simulink model "sequentialProcessorNarenKolli"  (R2018b)
settings: Solver=VariableStepAuto  StartTime=0.0  StopTime=10  RelTol=1e-3
libraries: hdlsllib x172, simulink_extras x9
(part 1 of 4)
settings Model: Creator=User  LastModifiedBy=kolli
settings DataIOCC: ReturnWorkspaceOutputs=on

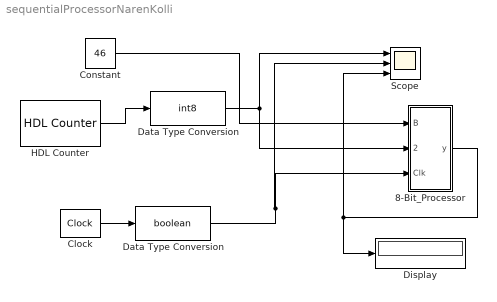
== system sequentialProcessorNarenKolli ==
  "8-Bit_Processor " : Subsystem
  "Clock " : simulink_extras/Flip Flops/Clock  period=1
  "Constant " : Constant  Value=46  OutDataTypeStr=uint8  SampleTime=1
  "Data Type Conversion " : DataTypeConversion  OutDataTypeStr=boolean
  "Data Type Conversion " : DataTypeConversion  OutDataTypeStr=int8
  "Display " : Display
  "HDL Counter " : hdlsllib/Sources/HDL Counter  CountType=Free running  CountInit=0  CountStep=1  CountMax=25  CountFromType=Initial value  CountFrom=0  CountResetPort=off  CountLoadPort=off  CountEnbPort=off  CountDirPort=off  CountDataType=Unsigned  CountWordLen=2  CountFracLen=0  CountSampTime=1
      settings: SourceProductName=Simulink
  "Scope " : Scope  NumInputPorts=3
  wires:
  "Constant "/1 -> "8-Bit_Processor "/1(B)
  "Data Type Conversion "/1 -> "Scope "/2, "8-Bit_Processor "/3("Clk ")
  "Clock "/1 -> "Data Type Conversion "/1
  "8-Bit_Processor "/1(y) -> "Scope "/3, "Display "/1
  "HDL Counter "/1 -> "Data Type Conversion "/1
  "Data Type Conversion "/1 -> "8-Bit_Processor "/2(Code), "Scope "/1

== system sequentialProcessorNarenKolli/8-Bit_Processor  ==
  B : Inport
  Code : Inport  Port=2
  "Clk " : Inport  Port=3
  8-Bit_Adder : Subsystem
  8-Bit_Bitwise_AND : Subsystem
  8-Bit_Multiplier : Subsystem
  8-Bit_Subtractor : Subsystem
  8-bit 4-to-1 MUX : Subsystem
  8-bit Register : Subsystem
  y : Outport  VectorParamsAs1DForOutWhenUnconnected=on
  wires:
  Code/1 -> 8-bit 4-to-1 MUX/1(s)
  8-bit 4-to-1 MUX/1(Y) -> 8-bit Register/1(Data_In), y/1
  8-Bit_Bitwise_AND/1(Y) -> 8-bit 4-to-1 MUX/5(D(11))
  "Clk "/1 -> 8-bit Register/2(Clk)
  8-Bit_Subtractor/1(Diff) -> 8-bit 4-to-1 MUX/4(C(10))
  8-bit Register/1(Y) -> 8-Bit_Bitwise_AND/2(B), 8-Bit_Subtractor/1(A), 8-Bit_Adder/2("B "), 8-Bit_Multiplier/2(B)
  8-Bit_Adder/1(Sum) -> 8-bit 4-to-1 MUX/2(A(00))
  8-Bit_Multiplier/1(Product) -> 8-bit 4-to-1 MUX/3(B(01))
  B/1 -> 8-Bit_Multiplier/1(A), 8-Bit_Adder/1("A "), 8-Bit_Bitwise_AND/1(A), 8-Bit_Subtractor/2(B)

== system sequentialProcessorNarenKolli/8-Bit_Processor /8-Bit_Adder ==
  "A " : Inport  OutDataTypeStr=uint8
  "B " : Inport  Port=2  OutDataTypeStr=uint8
  "Bit Concat " : hdlsllib/Logic and Bit Operations/Bit Concat  numInputs=8
      settings: SourceProductName=HDL Coder  SourceProductBaseCode=HD
  Constant2 : Constant  Value=0  OutDataTypeStr=boolean
  "Full Adder 0 " : Subsystem
  "Full Adder 1 " : Subsystem
  "Full Adder 2 " : Subsystem
  "Full Adder 3 " : Subsystem
  "Full Adder 4 " : Subsystem
  "Full Adder 5 " : Subsystem
  "Full Adder 6 " : Subsystem
  "Full Adder 7 " : Subsystem
  "Slicer1 " : Subsystem
  "Slicer2 " : Subsystem
  Sum : Outport  OutDataTypeStr=uint8
  wires:
  "Slicer1 "/3(Y5) -> "Full Adder 2 "/1(X)
  "Slicer2 "/7(Y1) -> "Full Adder 6 "/2(Y)
  "Full Adder 0 "/1(S) -> "Bit Concat "/1
  "Slicer1 "/1(Y7) -> "Full Adder 0 "/1(X)
  "Full Adder 1 "/1(S) -> "Bit Concat "/2
  "Slicer1 "/2(Y6) -> "Full Adder 1 "/1(X)
  "Slicer1 "/7(Y1) -> "Full Adder 6 "/1(X)
  "Slicer2 "/3(Y5) -> "Full Adder 2 "/2(Y)
  "Full Adder 5 "/1(S) -> "Bit Concat "/6
  "Slicer2 "/4(Y4) -> "Full Adder 3 "/2(Y)
  "Full Adder 3 "/2(C) -> "Full Adder 2 "/3(Z)
  "Full Adder 6 "/2(C) -> "Full Adder 5 "/3(Z)
  "Slicer1 "/6(Y2) -> "Full Adder 5 "/1(X)
  "B "/1 -> "Slicer2 "/1(X)
  "Slicer1 "/8(Y0) -> "Full Adder 7 "/1(X)
  "Full Adder 7 "/1(S) -> "Bit Concat "/8
  "Full Adder 6 "/1(S) -> "Bit Concat "/7
  "Slicer2 "/1(Y7) -> "Full Adder 0 "/2(Y)
  "Full Adder 3 "/1(S) -> "Bit Concat "/4
  "Full Adder 4 "/1(S) -> "Bit Concat "/5
  "Full Adder 2 "/2(C) -> "Full Adder 1 "/3(Z)
  "Slicer2 "/8(Y0) -> "Full Adder 7 "/2(Y)
  "Slicer2 "/2(Y6) -> "Full Adder 1 "/2(Y)
  "Full Adder 2 "/1(S) -> "Bit Concat "/3
  "Full Adder 7 "/2(C) -> "Full Adder 6 "/3(Z)
  Constant2/1 -> "Full Adder 7 "/3(Z)
  "Full Adder 1 "/2(C) -> "Full Adder 0 "/3(Z)
  "Full Adder 4 "/2(C) -> "Full Adder 3 "/3(Z)
  "Bit Concat "/1 -> Sum/1
  "Slicer2 "/6(Y2) -> "Full Adder 5 "/2(Y)
  "Slicer2 "/5(Y3) -> "Full Adder 4 "/2(Y)
  "A "/1 -> "Slicer1 "/1(X)
  "Full Adder 5 "/2(C) -> "Full Adder 4 "/3(Z)
  "Slicer1 "/4(Y4) -> "Full Adder 3 "/1(X)
  "Slicer1 "/5(Y3) -> "Full Adder 4 "/1(X)

== system sequentialProcessorNarenKolli/8-Bit_Processor /8-Bit_Bitwise_AND ==
  A : Inport
  B : Inport  Port=2
  AND{,1..7} (8 alike) : Logic  AllPortsSameDT=off  OutDataTypeStr=boolean
  Bit Concat Block : hdlsllib/Logic and Bit Operations/Bit Concat  numInputs=8
      settings: SourceProductName=HDL Coder  SourceProductBaseCode=HD
  First Bit Slicer : Subsystem
  Second Bit Slicer : Subsystem
  Y : Outport
  wires:
  AND2/1 -> Bit Concat Block/6
  AND4/1 -> Bit Concat Block/4
  Bit Concat Block/1 -> Y/1
  AND7/1 -> Bit Concat Block/1
  AND3/1 -> Bit Concat Block/5
  AND6/1 -> Bit Concat Block/2
  First Bit Slicer/6(Y2) -> AND2/1
  Second Bit Slicer/6(Y2) -> AND2/2
  Second Bit Slicer/1(Y7) -> AND7/2
  Second Bit Slicer/8(Y0) -> AND/2
  AND1/1 -> Bit Concat Block/7
  First Bit Slicer/7(Y1) -> AND1/1
  A/1 -> First Bit Slicer/1(X)
  B/1 -> Second Bit Slicer/1(X)
  Second Bit Slicer/7(Y1) -> AND1/2
  AND5/1 -> Bit Concat Block/3
  First Bit Slicer/8(Y0) -> AND/1
  First Bit Slicer/5(Y3) -> AND3/1
  AND/1 -> Bit Concat Block/8
  Second Bit Slicer/5(Y3) -> AND3/2
  Second Bit Slicer/4(Y4) -> AND4/2
  Second Bit Slicer/3(Y5) -> AND5/2
  First Bit Slicer/3(Y5) -> AND5/1
  First Bit Slicer/2(Y6) -> AND6/1
  First Bit Slicer/4(Y4) -> AND4/1
  Second Bit Slicer/2(Y6) -> AND6/2
  First Bit Slicer/1(Y7) -> AND7/1

== system sequentialProcessorNarenKolli/8-Bit_Processor /8-Bit_Multiplier ==
  A : Inport  OutDataTypeStr=uint8
  B : Inport  Port=2  OutDataTypeStr=uint8
  "First 4x4 Multiplier " : Subsystem
  First 8-Bit_Adder : Subsystem
  "First Bit Concat " : hdlsllib/Logic and Bit Operations/Bit Concat  numInputs=8
      settings: SourceProductName=HDL Coder  SourceProductBaseCode=HD
  First Constant : Constant  Value=0  OutDataTypeStr=boolean
  "First Slicer " : Subsystem
  "Fourth Bit Concat " : hdlsllib/Logic and Bit Operations/Bit Concat  numInputs=8
      settings: SourceProductName=HDL Coder  SourceProductBaseCode=HD
  Fourth Constant : Constant  Value=0  OutDataTypeStr=boolean
  Second 4x4 Multiplier : Subsystem
  Second 8-Bit_Adder1 : Subsystem
  "Second Bit Concat " : hdlsllib/Logic and Bit Operations/Bit Concat  numInputs=8
      settings: SourceProductName=HDL Coder  SourceProductBaseCode=HD
  Second Constant : Constant  Value=0  OutDataTypeStr=boolean
  Second Slicer : Subsystem
  Third Slicer : Subsystem
  Third 4x4 Multiplier : Subsystem
  "Third Bit Concat " : hdlsllib/Logic and Bit Operations/Bit Concat  numInputs=8
      settings: SourceProductName=HDL Coder  SourceProductBaseCode=HD
  Third Constant : Constant  Value=0  OutDataTypeStr=boolean
  Product : Outport  OutDataTypeStr=uint8
  wires:
  A/1 -> "First Slicer "/1(X)
  "First Slicer "/6(Y2) -> Third 4x4 Multiplier/2(A2), Second 4x4 Multiplier/2(A2)
  Third 4x4 Multiplier/6(Bit-2) -> "Fourth Bit Concat "/6
  "First Slicer "/5(Y3) -> Third 4x4 Multiplier/1(A3), Second 4x4 Multiplier/1(A3)
  Second 4x4 Multiplier/8(Bit-0) -> "Second Bit Concat "/8
  "First 4x4 Multiplier "/6(Bit-2) -> "First Bit Concat "/6
  "Second Bit Concat "/1 -> First 8-Bit_Adder/2(B)
  "First Slicer "/1(Y7) -> "First 4x4 Multiplier "/1(A3)
  Second Slicer/4(Y4) -> Second 4x4 Multiplier/8(B0)
  Second Slicer/1(Y7) -> Second 4x4 Multiplier/5(B3)
  Second Slicer/6(Y2) -> "First 4x4 Multiplier "/6(B2), Third 4x4 Multiplier/6(B2)
  "First Slicer "/7(Y1) -> Third 4x4 Multiplier/3(A1), Second 4x4 Multiplier/3(A1)
  Second Slicer/7(Y1) -> "First 4x4 Multiplier "/7(B1), Third 4x4 Multiplier/7(B1)
  Third Slicer/5(Y3) -> "Fourth Bit Concat "/1
  "First Slicer "/8(Y0) -> Third 4x4 Multiplier/4(A0), Second 4x4 Multiplier/4(A0)
  "Third Bit Concat "/1 -> Second 8-Bit_Adder1/2(B)
  Third Slicer/8(Y0) -> "Fourth Bit Concat "/4
  First 8-Bit_Adder/1(Sum) -> Second 8-Bit_Adder1/1(A)
  Second Slicer/5(Y3) -> Third 4x4 Multiplier/5(B3), "First 4x4 Multiplier "/5(B3)
  "First Slicer "/2(Y6) -> "First 4x4 Multiplier "/2(A2)
  "First 4x4 Multiplier "/7(Bit-1) -> "First Bit Concat "/7
  Second Slicer/8(Y0) -> "First 4x4 Multiplier "/8(B0), Third 4x4 Multiplier/8(B0)
  Third 4x4 Multiplier/1(Bit-7) -> "Third Bit Concat "/5
  Third Constant/1 -> "Third Bit Concat "/3
  "First Slicer "/3(Y5) -> "First 4x4 Multiplier "/3(A1)
  "First Slicer "/4(Y4) -> "First 4x4 Multiplier "/4(A0)
  First Constant/1 -> "Third Bit Concat "/1
  Second Slicer/3(Y5) -> Second 4x4 Multiplier/7(B1)
  Second Slicer/2(Y6) -> Second 4x4 Multiplier/6(B2)
  Third 4x4 Multiplier/8(Bit-0) -> "Fourth Bit Concat "/8
  "First Bit Concat "/1 -> First 8-Bit_Adder/1(A)
  "Fourth Bit Concat "/1 -> Product/1
  Third 4x4 Multiplier/5(Bit-3) -> "Fourth Bit Concat "/5
  Second 4x4 Multiplier/7(Bit-1) -> "Second Bit Concat "/7
  Third Slicer/7(Y1) -> "Fourth Bit Concat "/3
  Second 4x4 Multiplier/3(Bit-5) -> "Second Bit Concat "/3
  Third 4x4 Multiplier/7(Bit-1) -> "Fourth Bit Concat "/7
  Second 8-Bit_Adder1/1(Sum) -> Third Slicer/1(X)
  B/1 -> Second Slicer/1(X)
  Third Slicer/6(Y2) -> "Fourth Bit Concat "/2
  "First 4x4 Multiplier "/2(Bit-6) -> "First Bit Concat "/2
  "First 4x4 Multiplier "/4(Bit-4) -> "First Bit Concat "/4
  "First 4x4 Multiplier "/8(Bit-0) -> "First Bit Concat "/8
  Second 4x4 Multiplier/6(Bit-2) -> "Second Bit Concat "/6
  Second 4x4 Multiplier/5(Bit-3) -> "Second Bit Concat "/5
  Fourth Constant/1 -> "Third Bit Concat "/4
  Second 4x4 Multiplier/4(Bit-4) -> "Second Bit Concat "/4
  "First 4x4 Multiplier "/3(Bit-5) -> "First Bit Concat "/3
  "First 4x4 Multiplier "/5(Bit-3) -> "First Bit Concat "/5
  "First 4x4 Multiplier "/1(Bit-7) -> "First Bit Concat "/1
  Second 4x4 Multiplier/2(Bit-6) -> "Second Bit Concat "/2
  Second Constant/1 -> "Third Bit Concat "/2
  Third 4x4 Multiplier/4(Bit-4) -> "Third Bit Concat "/8
  Third 4x4 Multiplier/3(Bit-5) -> "Third Bit Concat "/7
  Third 4x4 Multiplier/2(Bit-6) -> "Third Bit Concat "/6
  Second 4x4 Multiplier/1(Bit-7) -> "Second Bit Concat "/1

== system sequentialProcessorNarenKolli/8-Bit_Processor /8-Bit_Subtractor ==
  A : Inport  OutDataTypeStr=uint8
  B : Inport  Port=2  OutDataTypeStr=uint8
  Bit Concat : hdlsllib/Logic and Bit Operations/Bit Concat  numInputs=8
      settings: SourceProductName=HDL Coder  SourceProductBaseCode=HD
  Constant2 : Constant  OutDataTypeStr=boolean
  Full Adder 0 : Subsystem
  Full Adder 1 : Subsystem
  "Full Adder 2 " : Subsystem
  "Full Adder 3 " : Subsystem
  Full Adder 4 : Subsystem
  "Full Adder 5 " : Subsystem
  "Full Adder 6 " : Subsystem
  "Full Adder 7 " : Subsystem
  "NOT 0 " : Logic  Operator=NOT  AllPortsSameDT=off  OutDataTypeStr=boolean
  NOT {1..7} (7 alike) : Logic  Operator=NOT  AllPortsSameDT=off  OutDataTypeStr=boolean
  "Slicer 1 " : Subsystem
  "Slicer 2 " : Subsystem
  Diff : Outport  OutDataTypeStr=uint8
  wires:
  "Slicer 1 "/3(Y5) -> "Full Adder 2 "/1(X)
  "Slicer 2 "/7(Y1) -> NOT 6/1
  Full Adder 0/1(S) -> Bit Concat/1
  "Slicer 1 "/1(Y7) -> Full Adder 0/1(X)
  Full Adder 1/1(S) -> Bit Concat/2
  "Slicer 1 "/2(Y6) -> Full Adder 1/1(X)
  "Slicer 1 "/7(Y1) -> "Full Adder 6 "/1(X)
  "Slicer 2 "/3(Y5) -> NOT 2/1
  "Full Adder 5 "/1(S) -> Bit Concat/6
  "Slicer 2 "/4(Y4) -> NOT 3/1
  "Full Adder 3 "/2(C) -> "Full Adder 2 "/3(Z)
  "Full Adder 6 "/2(C) -> "Full Adder 5 "/3(Z)
  "Slicer 1 "/6(Y2) -> "Full Adder 5 "/1(X)
  B/1 -> "Slicer 2 "/1(X)
  "Slicer 1 "/8(Y0) -> "Full Adder 7 "/1(X)
  "Full Adder 7 "/1(S) -> Bit Concat/8
  "Full Adder 6 "/1(S) -> Bit Concat/7
  "NOT 0 "/1 -> Full Adder 0/2(Y)
  "Full Adder 3 "/1(S) -> Bit Concat/4
  Full Adder 4/1(S) -> Bit Concat/5
  "Full Adder 2 "/2(C) -> Full Adder 1/3(Z)
  "Slicer 2 "/8(Y0) -> NOT 7/1
  "Slicer 2 "/2(Y6) -> NOT 1/1
  "Full Adder 2 "/1(S) -> Bit Concat/3
  "Full Adder 7 "/2(C) -> "Full Adder 6 "/3(Z)
  Constant2/1 -> "Full Adder 7 "/3(Z)
  Full Adder 1/2(C) -> Full Adder 0/3(Z)
  Full Adder 4/2(C) -> "Full Adder 3 "/3(Z)
  Bit Concat/1 -> Diff/1
  "Slicer 2 "/6(Y2) -> NOT 5/1
  "Slicer 2 "/5(Y3) -> NOT 4/1
  A/1 -> "Slicer 1 "/1(X)
  "Full Adder 5 "/2(C) -> Full Adder 4/3(Z)
  "Slicer 1 "/4(Y4) -> "Full Adder 3 "/1(X)
  "Slicer 1 "/5(Y3) -> Full Adder 4/1(X)
  NOT 1/1 -> Full Adder 1/2(Y)
  "Slicer 2 "/1(Y7) -> "NOT 0 "/1
  NOT 2/1 -> "Full Adder 2 "/2(Y)
  NOT 3/1 -> "Full Adder 3 "/2(Y)
  NOT 4/1 -> Full Adder 4/2(Y)
  NOT 5/1 -> "Full Adder 5 "/2(Y)
  NOT 6/1 -> "Full Adder 6 "/2(Y)
  NOT 7/1 -> "Full Adder 7 "/2(Y)

== system sequentialProcessorNarenKolli/8-Bit_Processor /8-bit 4-to-1 MUX ==
  s : Inport
  A(00) : Inport  Port=2
  B(01) : Inport  Port=3
  C(10) : Inport  Port=4
  D(11) : Inport  Port=5
  4 x 1 MUX : Subsystem
  4 x 1 MUX1 : Subsystem
  4 x 1 MUX2 : Subsystem
  4 x 1 MUX3 : Subsystem
  4 x 1 MUX4 : Subsystem
  4 x 1 MUX5 : Subsystem
  4 x 1 MUX6 : Subsystem
  4 x 1 MUX7 : Subsystem
  Bit Concat : hdlsllib/Logic and Bit Operations/Bit Concat  numInputs=8
      settings: SourceProductName=Simulink
  Slicer : Subsystem
  Slicer1 : Subsystem
  Slicer2 : Subsystem
  Slicer3 : Subsystem
  Y : Outport  VectorParamsAs1DForOutWhenUnconnected=on
  wires:
  Slicer1/7(Y6) -> 4 x 1 MUX6/4(x1)
  Slicer3/8(Y7) -> 4 x 1 MUX7/5(x3)
  Slicer1/8(Y7) -> 4 x 1 MUX7/4(x1)
  s/1 -> 4 x 1 MUX/1(s), 4 x 1 MUX6/1(s), 4 x 1 MUX7/1(s), 4 x 1 MUX5/1(s), 4 x 1 MUX4/1(s), 4 x 1 MUX3/1(s), 4 x 1 MUX2/1(s), 4 x 1 MUX1/1(s)
  A(00)/1 -> Slicer/1(In1)
  Slicer/8(Y7) -> 4 x 1 MUX7/2("x0 ")
  Slicer2/1(Y0) -> 4 x 1 MUX/3(x2)
  4 x 1 MUX5/1(y) -> Bit Concat/3
  Bit Concat/1 -> Y/1
  Slicer3/2(Y1) -> 4 x 1 MUX1/5(x3)
  Slicer/7(Y6) -> 4 x 1 MUX6/2("x0 ")
  D(11)/1 -> Slicer3/1(In1)
  Slicer2/6(Y5) -> 4 x 1 MUX5/3(x2)
  4 x 1 MUX7/1(y) -> Bit Concat/1
  Slicer3/3(Y2) -> 4 x 1 MUX2/5(x3)
  Slicer3/5(Y4) -> 4 x 1 MUX4/5(x3)
  Slicer/6(Y5) -> 4 x 1 MUX5/2("x0 ")
  B(01)/1 -> Slicer1/1(In1)
  Slicer3/6(Y5) -> 4 x 1 MUX5/5(x3)
  Slicer3/7(Y6) -> 4 x 1 MUX6/5(x3)
  Slicer2/5(Y4) -> 4 x 1 MUX4/3(x2)
  Slicer2/2(Y1) -> 4 x 1 MUX1/3(x2)
  4 x 1 MUX/1(y) -> Bit Concat/8
  4 x 1 MUX4/1(y) -> Bit Concat/4
  4 x 1 MUX3/1(y) -> Bit Concat/5
  4 x 1 MUX6/1(y) -> Bit Concat/2
  Slicer1/3(Y2) -> 4 x 1 MUX2/4(x1)
  Slicer2/3(Y2) -> 4 x 1 MUX2/3(x2)
  Slicer1/6(Y5) -> 4 x 1 MUX5/4(x1)
  Slicer1/4(Y3) -> 4 x 1 MUX3/4(x1)
  Slicer2/8(Y7) -> 4 x 1 MUX7/3(x2)
  Slicer/2(Y1) -> 4 x 1 MUX1/2("x0 ")
  Slicer/4(Y3) -> 4 x 1 MUX3/2("x0 ")
  Slicer2/4(Y3) -> 4 x 1 MUX3/3(x2)
  Slicer3/1(Y0) -> 4 x 1 MUX/5(x3)
  Slicer3/4(Y3) -> 4 x 1 MUX3/5(x3)
  Slicer1/5(Y4) -> 4 x 1 MUX4/4(x1)
  Slicer/3(Y2) -> 4 x 1 MUX2/2("x0 ")
  Slicer/5(Y4) -> 4 x 1 MUX4/2("x0 ")
  Slicer2/7(Y6) -> 4 x 1 MUX6/3(x2)
  4 x 1 MUX1/1(y) -> Bit Concat/7
  Slicer1/2(Y1) -> 4 x 1 MUX1/4(x1)
  C(10)/1 -> Slicer2/1(In1)
  Slicer1/1(Y0) -> 4 x 1 MUX/4(x1)
  4 x 1 MUX2/1(y) -> Bit Concat/6
  Slicer/1(Y0) -> 4 x 1 MUX/2("x0 ")

== system sequentialProcessorNarenKolli/8-Bit_Processor /8-bit Register ==
  Data_In : Inport
  Clk : Inport  Port=2
  Bit Concat : hdlsllib/Logic and Bit Operations/Bit Concat  numInputs=8
      settings: SourceProductName=Simulink
  Constant : Constant  OutDataTypeStr=boolean  SampleTime=1
  D Flip-Flop{,1..7} (8 alike) : simulink_extras/Flip Flops/D Flip-Flop
      settings: SourceProductName=Simulink
  Slicer : Subsystem
  Terminator{,1..7} (8 alike) : Terminator
  Y : Outport  VectorParamsAs1DForOutWhenUnconnected=on
  wires:
  Constant/1 -> D Flip-Flop4/3, D Flip-Flop7/3, D Flip-Flop6/3, D Flip-Flop5/3, D Flip-Flop3/3, D Flip-Flop2/3, D Flip-Flop1/3, D Flip-Flop/3
  Clk/1 -> D Flip-Flop6/2, D Flip-Flop7/2, D Flip-Flop5/2, D Flip-Flop4/2, D Flip-Flop3/2, D Flip-Flop2/2, D Flip-Flop1/2, D Flip-Flop/2
  D Flip-Flop5/1 -> Bit Concat/3
  Slicer/8(Y7) -> D Flip-Flop7/1
  D Flip-Flop1/2 -> Terminator1/1
  D Flip-Flop/1 -> Bit Concat/8
  D Flip-Flop1/1 -> Bit Concat/7
  Data_In/1 -> Slicer/1(In1)
  D Flip-Flop2/2 -> Terminator2/1
  Bit Concat/1 -> Y/1
  Slicer/7(Y6) -> D Flip-Flop6/1
  D Flip-Flop7/1 -> Bit Concat/1
  D Flip-Flop6/2 -> Terminator6/1
  D Flip-Flop4/2 -> Terminator4/1
  Slicer/4(Y3) -> D Flip-Flop3/1
  D Flip-Flop3/2 -> Terminator3/1
  D Flip-Flop2/1 -> Bit Concat/6
  Slicer/2(Y1) -> D Flip-Flop1/1
  D Flip-Flop/2 -> Terminator/1
  D Flip-Flop4/1 -> Bit Concat/4
  D Flip-Flop7/2 -> Terminator7/1
  D Flip-Flop3/1 -> Bit Concat/5
  Slicer/5(Y4) -> D Flip-Flop4/1
  Slicer/1(Y0) -> D Flip-Flop/1
  D Flip-Flop5/2 -> Terminator5/1
  Slicer/6(Y5) -> D Flip-Flop5/1
  Slicer/3(Y2) -> D Flip-Flop2/1
  D Flip-Flop6/1 -> Bit Concat/2

== system sequentialProcessorNarenKolli/8-Bit_Processor /8-Bit_Adder/Full Adder 0  ==
  X : Inport
  Y : Inport  Port=2
  Z : Inport  Port=3
  Half Adder : Subsystem
  Half Adder1 : Subsystem
  OR : Logic  Operator=OR  AllPortsSameDT=off  OutDataTypeStr=boolean
  S : Outport
  C : Outport  Port=2
  wires:
  Half Adder/2(Carry) -> OR/2
  OR/1 -> C/1
  Z/1 -> Half Adder1/2(B)
  X/1 -> Half Adder/1(A)
  Half Adder1/1(Sum) -> S/1
  Half Adder/1(Sum) -> Half Adder1/1(A)
  Y/1 -> Half Adder/2(B)
  Half Adder1/2(Carry) -> OR/1

== system sequentialProcessorNarenKolli/8-Bit_Processor /8-Bit_Adder/Full Adder 1  ==
  X : Inport
  Y : Inport  Port=2
  Z : Inport  Port=3
  Half Adder : Subsystem
  Half Adder1 : Subsystem
  OR : Logic  Operator=OR  AllPortsSameDT=off  OutDataTypeStr=boolean
  S : Outport
  C : Outport  Port=2
  wires:
  Half Adder/2(Carry) -> OR/2
  OR/1 -> C/1
  Z/1 -> Half Adder1/2(B)
  X/1 -> Half Adder/1(A)
  Half Adder1/1(Sum) -> S/1
  Half Adder/1(Sum) -> Half Adder1/1(A)
  Y/1 -> Half Adder/2(B)
  Half Adder1/2(Carry) -> OR/1

== system sequentialProcessorNarenKolli/8-Bit_Processor /8-Bit_Adder/Full Adder 2  ==
  X : Inport
  Y : Inport  Port=2
  Z : Inport  Port=3
  Half Adder : Subsystem
  Half Adder1 : Subsystem
  OR : Logic  Operator=OR  AllPortsSameDT=off  OutDataTypeStr=boolean
  S : Outport
  C : Outport  Port=2
  wires:
  Half Adder/2(Carry) -> OR/2
  OR/1 -> C/1
  Z/1 -> Half Adder1/2(B)
  X/1 -> Half Adder/1(A)
  Half Adder1/1(Sum) -> S/1
  Half Adder/1(Sum) -> Half Adder1/1(A)
  Y/1 -> Half Adder/2(B)
  Half Adder1/2(Carry) -> OR/1

== system sequentialProcessorNarenKolli/8-Bit_Processor /8-Bit_Adder/Full Adder 3  ==
  X : Inport
  Y : Inport  Port=2
  Z : Inport  Port=3
  Half Adder : Subsystem
  Half Adder1 : Subsystem
  OR : Logic  Operator=OR  AllPortsSameDT=off  OutDataTypeStr=boolean
  S : Outport
  C : Outport  Port=2
  wires:
  Half Adder/2(Carry) -> OR/2
  OR/1 -> C/1
  Z/1 -> Half Adder1/2(B)
  X/1 -> Half Adder/1(A)
  Half Adder1/1(Sum) -> S/1
  Half Adder/1(Sum) -> Half Adder1/1(A)
  Y/1 -> Half Adder/2(B)
  Half Adder1/2(Carry) -> OR/1

== system sequentialProcessorNarenKolli/8-Bit_Processor /8-Bit_Adder/Full Adder 4  ==
  X : Inport
  Y : Inport  Port=2
  Z : Inport  Port=3
  Half Adder : Subsystem
  Half Adder1 : Subsystem
  OR : Logic  Operator=OR  AllPortsSameDT=off  OutDataTypeStr=boolean
  S : Outport
  C : Outport  Port=2
  wires:
  Half Adder/2(Carry) -> OR/2
  OR/1 -> C/1
  Z/1 -> Half Adder1/2(B)
  X/1 -> Half Adder/1(A)
  Half Adder1/1(Sum) -> S/1
  Half Adder/1(Sum) -> Half Adder1/1(A)
  Y/1 -> Half Adder/2(B)
  Half Adder1/2(Carry) -> OR/1

== system sequentialProcessorNarenKolli/8-Bit_Processor /8-Bit_Adder/Full Adder 5  ==
  X : Inport
  Y : Inport  Port=2
  Z : Inport  Port=3
  Half Adder : Subsystem
  Half Adder1 : Subsystem
  OR : Logic  Operator=OR  AllPortsSameDT=off  OutDataTypeStr=boolean
  S : Outport
  C : Outport  Port=2
  wires:
  Half Adder/2(Carry) -> OR/2
  OR/1 -> C/1
  Z/1 -> Half Adder1/2(B)
  X/1 -> Half Adder/1(A)
  Half Adder1/1(Sum) -> S/1
  Half Adder/1(Sum) -> Half Adder1/1(A)
  Y/1 -> Half Adder/2(B)
  Half Adder1/2(Carry) -> OR/1

== system sequentialProcessorNarenKolli/8-Bit_Processor /8-Bit_Adder/Full Adder 6  ==
  X : Inport
  Y : Inport  Port=2
  Z : Inport  Port=3
  Half Adder : Subsystem
  Half Adder1 : Subsystem
  OR : Logic  Operator=OR  AllPortsSameDT=off  OutDataTypeStr=boolean
  S : Outport
  C : Outport  Port=2
  wires:
  Half Adder/2(Carry) -> OR/2
  OR/1 -> C/1
  Z/1 -> Half Adder1/2(B)
  X/1 -> Half Adder/1(A)
  Half Adder1/1(Sum) -> S/1
  Half Adder/1(Sum) -> Half Adder1/1(A)
  Y/1 -> Half Adder/2(B)
  Half Adder1/2(Carry) -> OR/1

== system sequentialProcessorNarenKolli/8-Bit_Processor /8-Bit_Adder/Full Adder 7  ==
  X : Inport
  Y : Inport  Port=2
  Z : Inport  Port=3
  Half Adder : Subsystem
  Half Adder1 : Subsystem
  OR : Logic  Operator=OR  AllPortsSameDT=off  OutDataTypeStr=boolean
  S : Outport
  C : Outport  Port=2
  wires:
  Half Adder/2(Carry) -> OR/2
  OR/1 -> C/1
  Z/1 -> Half Adder1/2(B)
  X/1 -> Half Adder/1(A)
  Half Adder1/1(Sum) -> S/1
  Half Adder/1(Sum) -> Half Adder1/1(A)
  Y/1 -> Half Adder/2(B)
  Half Adder1/2(Carry) -> OR/1

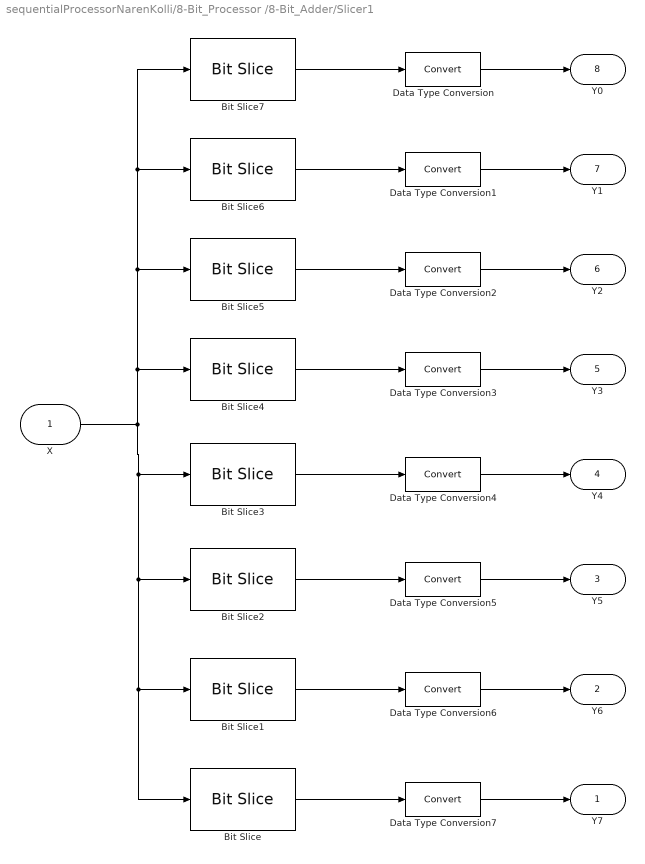
== system sequentialProcessorNarenKolli/8-Bit_Processor /8-Bit_Adder/Slicer1  ==
  X : Inport  OutDataTypeStr=uint8  SampleTime=1
  Bit Slice : hdlsllib/Logic and Bit Operations/Bit Slice  lidx=7  ridx=7
  Bit Slice1 : hdlsllib/Logic and Bit Operations/Bit Slice  lidx=6  ridx=6
  Bit Slice2 : hdlsllib/Logic and Bit Operations/Bit Slice  lidx=5  ridx=5
  Bit Slice3 : hdlsllib/Logic and Bit Operations/Bit Slice  lidx=4  ridx=4
  Bit Slice4 : hdlsllib/Logic and Bit Operations/Bit Slice  lidx=3  ridx=3
  Bit Slice5 : hdlsllib/Logic and Bit Operations/Bit Slice  lidx=2  ridx=2
  Bit Slice6 : hdlsllib/Logic and Bit Operations/Bit Slice  lidx=1  ridx=1
  Bit Slice7 : hdlsllib/Logic and Bit Operations/Bit Slice  lidx=0  ridx=0
  Data Type Conversion{,1..7} (8 alike) : DataTypeConversion
  Y7 : Outport
  Y6 : Outport  Port=2
  Y5 : Outport  Port=3
  Y4 : Outport  Port=4
  Y3 : Outport  Port=5
  Y2 : Outport  Port=6
  Y1 : Outport  Port=7
  Y0 : Outport  Port=8
  wires:
  Data Type Conversion4/1 -> Y4/1
  Bit Slice3/1 -> Data Type Conversion4/1
  X/1 -> Bit Slice3/1, Bit Slice2/1, Bit Slice1/1, Bit Slice/1, Bit Slice4/1, Bit Slice5/1, Bit Slice6/1, Bit Slice7/1
  Bit Slice1/1 -> Data Type Conversion6/1
  Data Type Conversion1/1 -> Y1/1
  Bit Slice6/1 -> Data Type Conversion1/1
  Bit Slice5/1 -> Data Type Conversion2/1
  Bit Slice2/1 -> Data Type Conversion5/1
  Data Type Conversion/1 -> Y0/1
  Bit Slice4/1 -> Data Type Conversion3/1
  Bit Slice/1 -> Data Type Conversion7/1
  Data Type Conversion7/1 -> Y7/1
  Bit Slice7/1 -> Data Type Conversion/1
  Data Type Conversion3/1 -> Y3/1
  Data Type Conversion5/1 -> Y5/1
  Data Type Conversion6/1 -> Y6/1
  Data Type Conversion2/1 -> Y2/1

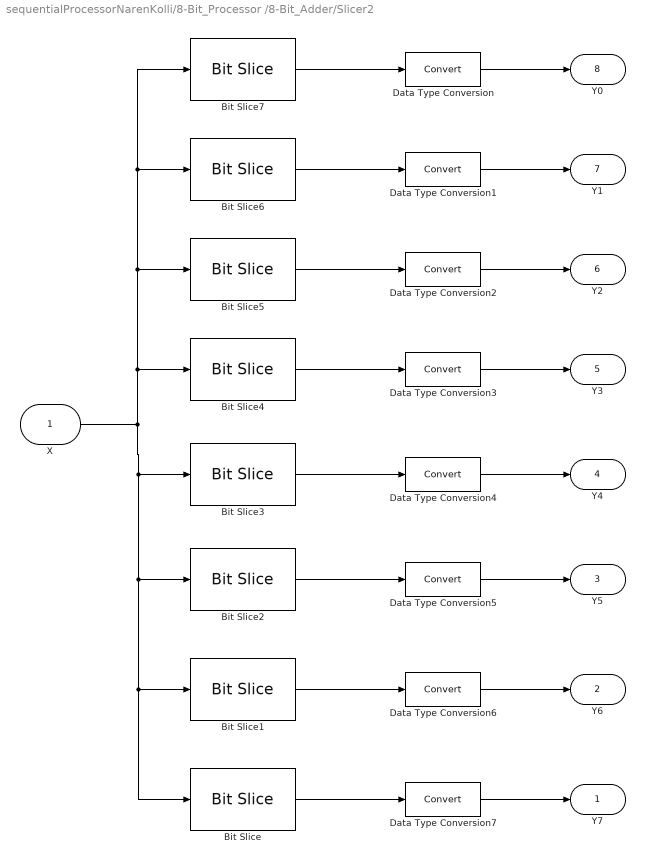
== system sequentialProcessorNarenKolli/8-Bit_Processor /8-Bit_Adder/Slicer2  ==
  X : Inport  OutDataTypeStr=uint8  SampleTime=1
  Bit Slice : hdlsllib/Logic and Bit Operations/Bit Slice  lidx=7  ridx=7
  Bit Slice1 : hdlsllib/Logic and Bit Operations/Bit Slice  lidx=6  ridx=6
  Bit Slice2 : hdlsllib/Logic and Bit Operations/Bit Slice  lidx=5  ridx=5
  Bit Slice3 : hdlsllib/Logic and Bit Operations/Bit Slice  lidx=4  ridx=4
  Bit Slice4 : hdlsllib/Logic and Bit Operations/Bit Slice  lidx=3  ridx=3
  Bit Slice5 : hdlsllib/Logic and Bit Operations/Bit Slice  lidx=2  ridx=2
  Bit Slice6 : hdlsllib/Logic and Bit Operations/Bit Slice  lidx=1  ridx=1
  Bit Slice7 : hdlsllib/Logic and Bit Operations/Bit Slice  lidx=0  ridx=0
  Data Type Conversion{,1..7} (8 alike) : DataTypeConversion
  Y7 : Outport
  Y6 : Outport  Port=2
  Y5 : Outport  Port=3
  Y4 : Outport  Port=4
  Y3 : Outport  Port=5
  Y2 : Outport  Port=6
  Y1 : Outport  Port=7
  Y0 : Outport  Port=8
  wires:
  Data Type Conversion4/1 -> Y4/1
  Bit Slice3/1 -> Data Type Conversion4/1
  X/1 -> Bit Slice3/1, Bit Slice2/1, Bit Slice1/1, Bit Slice/1, Bit Slice4/1, Bit Slice5/1, Bit Slice6/1, Bit Slice7/1
  Bit Slice1/1 -> Data Type Conversion6/1
  Data Type Conversion1/1 -> Y1/1
  Bit Slice6/1 -> Data Type Conversion1/1
  Bit Slice5/1 -> Data Type Conversion2/1
  Bit Slice2/1 -> Data Type Conversion5/1
  Data Type Conversion/1 -> Y0/1
  Bit Slice4/1 -> Data Type Conversion3/1
  Bit Slice/1 -> Data Type Conversion7/1
  Data Type Conversion7/1 -> Y7/1
  Bit Slice7/1 -> Data Type Conversion/1
  Data Type Conversion3/1 -> Y3/1
  Data Type Conversion5/1 -> Y5/1
  Data Type Conversion6/1 -> Y6/1
  Data Type Conversion2/1 -> Y2/1

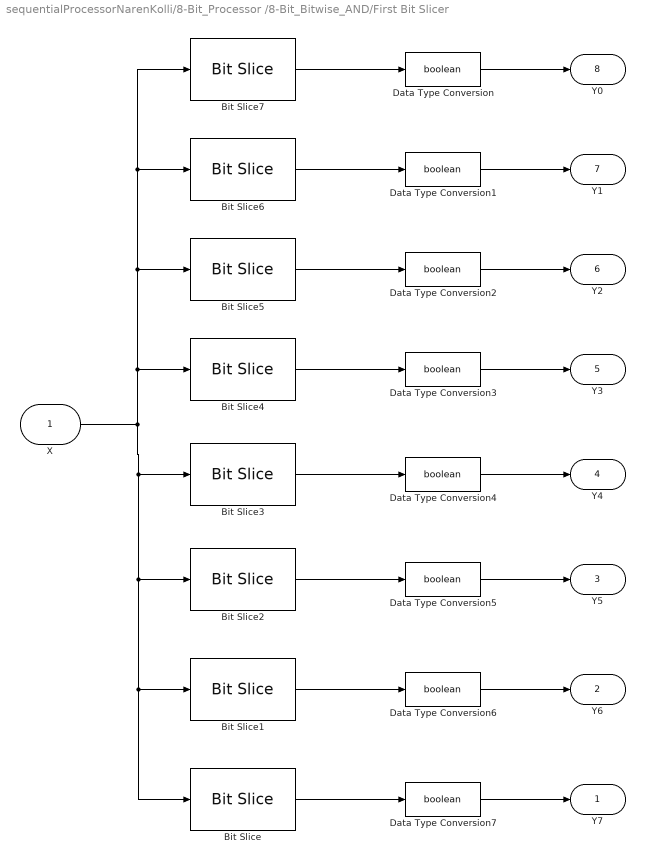
== system sequentialProcessorNarenKolli/8-Bit_Processor /8-Bit_Bitwise_AND/First Bit Slicer ==
  X : Inport  OutDataTypeStr=uint8  SampleTime=1
  Bit Slice : hdlsllib/Logic and Bit Operations/Bit Slice  lidx=7  ridx=7
  Bit Slice1 : hdlsllib/Logic and Bit Operations/Bit Slice  lidx=6  ridx=6
  Bit Slice2 : hdlsllib/Logic and Bit Operations/Bit Slice  lidx=5  ridx=5
  Bit Slice3 : hdlsllib/Logic and Bit Operations/Bit Slice  lidx=4  ridx=4
  Bit Slice4 : hdlsllib/Logic and Bit Operations/Bit Slice  lidx=3  ridx=3
  Bit Slice5 : hdlsllib/Logic and Bit Operations/Bit Slice  lidx=2  ridx=2
  Bit Slice6 : hdlsllib/Logic and Bit Operations/Bit Slice  lidx=1  ridx=1
  Bit Slice7 : hdlsllib/Logic and Bit Operations/Bit Slice  lidx=0  ridx=0
  Data Type Conversion{,1..7} (8 alike) : DataTypeConversion  OutDataTypeStr=boolean
  Y7 : Outport  OutDataTypeStr=boolean
  Y6 : Outport  Port=2  OutDataTypeStr=boolean
  Y5 : Outport  Port=3  OutDataTypeStr=boolean
  Y4 : Outport  Port=4  OutDataTypeStr=boolean
  Y3 : Outport  Port=5  OutDataTypeStr=boolean
  Y2 : Outport  Port=6  OutDataTypeStr=boolean
  Y1 : Outport  Port=7  OutDataTypeStr=boolean
  Y0 : Outport  Port=8  OutDataTypeStr=boolean
  wires:
  Data Type Conversion4/1 -> Y4/1
  Bit Slice3/1 -> Data Type Conversion4/1
  X/1 -> Bit Slice3/1, Bit Slice2/1, Bit Slice1/1, Bit Slice/1, Bit Slice4/1, Bit Slice5/1, Bit Slice6/1, Bit Slice7/1
  Bit Slice1/1 -> Data Type Conversion6/1
  Data Type Conversion1/1 -> Y1/1
  Bit Slice6/1 -> Data Type Conversion1/1
  Bit Slice5/1 -> Data Type Conversion2/1
  Bit Slice2/1 -> Data Type Conversion5/1
  Data Type Conversion/1 -> Y0/1
  Bit Slice4/1 -> Data Type Conversion3/1
  Bit Slice/1 -> Data Type Conversion7/1
  Data Type Conversion7/1 -> Y7/1
  Bit Slice7/1 -> Data Type Conversion/1
  Data Type Conversion3/1 -> Y3/1
  Data Type Conversion5/1 -> Y5/1
  Data Type Conversion6/1 -> Y6/1
  Data Type Conversion2/1 -> Y2/1

== system sequentialProcessorNarenKolli/8-Bit_Processor /8-Bit_Bitwise_AND/Second Bit Slicer ==
  X : Inport  OutDataTypeStr=uint8  SampleTime=1
  Bit Slice : hdlsllib/Logic and Bit Operations/Bit Slice  lidx=7  ridx=7
  Bit Slice1 : hdlsllib/Logic and Bit Operations/Bit Slice  lidx=6  ridx=6
  Bit Slice2 : hdlsllib/Logic and Bit Operations/Bit Slice  lidx=5  ridx=5
  Bit Slice3 : hdlsllib/Logic and Bit Operations/Bit Slice  lidx=4  ridx=4
  Bit Slice4 : hdlsllib/Logic and Bit Operations/Bit Slice  lidx=3  ridx=3
  Bit Slice5 : hdlsllib/Logic and Bit Operations/Bit Slice  lidx=2  ridx=2
  Bit Slice6 : hdlsllib/Logic and Bit Operations/Bit Slice  lidx=1  ridx=1
  Bit Slice7 : hdlsllib/Logic and Bit Operations/Bit Slice  lidx=0  ridx=0
  Data Type Conversion{,1..7} (8 alike) : DataTypeConversion  OutDataTypeStr=boolean
  Y7 : Outport  OutDataTypeStr=boolean
  Y6 : Outport  Port=2  OutDataTypeStr=boolean
  Y5 : Outport  Port=3  OutDataTypeStr=boolean
  Y4 : Outport  Port=4  OutDataTypeStr=boolean
  Y3 : Outport  Port=5  OutDataTypeStr=boolean
  Y2 : Outport  Port=6  OutDataTypeStr=boolean
  Y1 : Outport  Port=7  OutDataTypeStr=boolean
  Y0 : Outport  Port=8  OutDataTypeStr=boolean
  wires:
  Data Type Conversion4/1 -> Y4/1
  Bit Slice3/1 -> Data Type Conversion4/1
  X/1 -> Bit Slice3/1, Bit Slice2/1, Bit Slice1/1, Bit Slice/1, Bit Slice4/1, Bit Slice5/1, Bit Slice6/1, Bit Slice7/1
  Bit Slice1/1 -> Data Type Conversion6/1
  Data Type Conversion1/1 -> Y1/1
  Bit Slice6/1 -> Data Type Conversion1/1
  Bit Slice5/1 -> Data Type Conversion2/1
  Bit Slice2/1 -> Data Type Conversion5/1
  Data Type Conversion/1 -> Y0/1
  Bit Slice4/1 -> Data Type Conversion3/1
  Bit Slice/1 -> Data Type Conversion7/1
  Data Type Conversion7/1 -> Y7/1
  Bit Slice7/1 -> Data Type Conversion/1
  Data Type Conversion3/1 -> Y3/1
  Data Type Conversion5/1 -> Y5/1
  Data Type Conversion6/1 -> Y6/1
  Data Type Conversion2/1 -> Y2/1

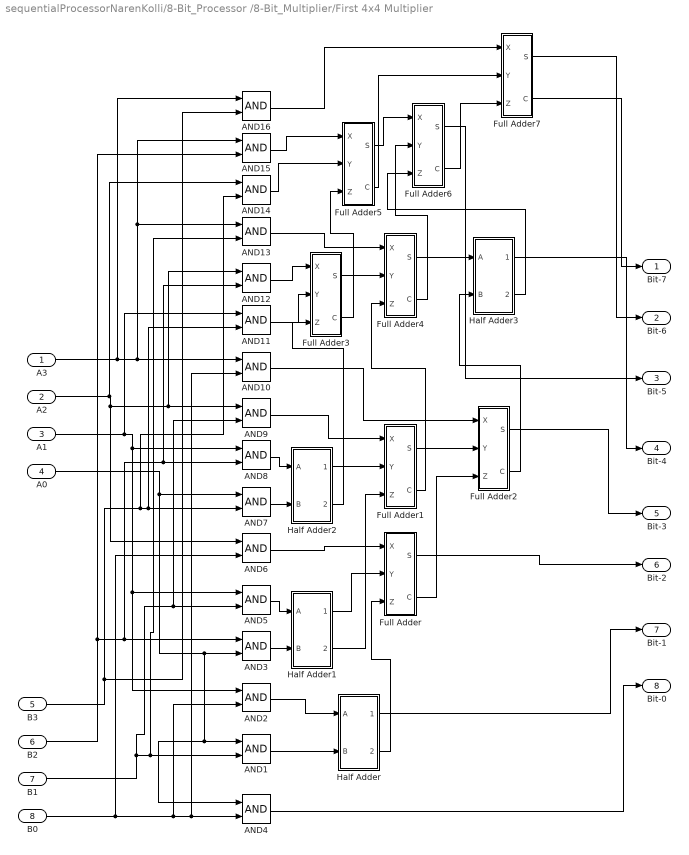
== system sequentialProcessorNarenKolli/8-Bit_Processor /8-Bit_Multiplier/First 4x4 Multiplier  ==
  A3 : Inport  OutDataTypeStr=boolean
  A2 : Inport  Port=2  OutDataTypeStr=boolean
  A1 : Inport  Port=3  OutDataTypeStr=boolean
  A0 : Inport  Port=4  OutDataTypeStr=boolean
  B3 : Inport  Port=5  OutDataTypeStr=boolean
  B2 : Inport  Port=6  OutDataTypeStr=boolean
  B1 : Inport  Port=7  OutDataTypeStr=boolean
  B0 : Inport  Port=8  OutDataTypeStr=boolean
  AND{1..16} (16 alike) : Logic  AllPortsSameDT=off  OutDataTypeStr=boolean
  Full Adder : Subsystem
  Full Adder1 : Subsystem
  Full Adder2 : Subsystem
  Full Adder3 : Subsystem
  Full Adder4 : Subsystem
  Full Adder5 : Subsystem
  Full Adder6 : Subsystem
  Full Adder7 : Subsystem
  Half Adder : Subsystem
  Half Adder1 : Subsystem
  Half Adder2 : Subsystem
  Half Adder3 : Subsystem
  Bit-7 : Outport  OutDataTypeStr=boolean
  Bit-6 : Outport  Port=2  OutDataTypeStr=boolean
  Bit-5 : Outport  Port=3  OutDataTypeStr=boolean
  Bit-4 : Outport  Port=4  OutDataTypeStr=boolean
  Bit-3 : Outport  Port=5  OutDataTypeStr=boolean
  Bit-2 : Outport  Port=6  OutDataTypeStr=boolean
  Bit-1 : Outport  Port=7  OutDataTypeStr=boolean
  Bit-0 : Outport  Port=8  OutDataTypeStr=boolean
  wires:
  AND4/1 -> Bit-0/1
  A0/1 -> AND7/1, AND3/2, AND4/1, AND1/1
  B0/1 -> AND6/2, AND10/2, AND4/2, AND2/2
  AND2/1 -> Half Adder/1(A)
  AND1/1 -> Half Adder/2(B)
  Half Adder/1(Sum) -> Bit-1/1
  B2/1 -> AND15/2, AND12/2, AND8/2, AND3/1
  AND3/1 -> Half Adder1/2(B)
  AND5/1 -> Half Adder1/1(A)
  A2/1 -> AND14/1, AND12/1, AND9/1, AND6/1
  Half Adder/2(Carry) -> Full Adder/3(Z)
  Half Adder1/1(Sum) -> Full Adder/2(Y)
  AND6/1 -> Full Adder/1(X)
  Full Adder/1(S) -> Bit-2/1
  B3/1 -> AND16/2, AND14/2, AND11/2, AND7/2
  B1/1 -> AND9/2, AND5/2, AND13/2, AND1/2
  A3/1 -> AND16/1, AND15/1, AND13/1, AND10/1
  AND7/1 -> Half Adder2/2(B)
  AND8/1 -> Half Adder2/1(A)
  Half Adder2/1(Sum) -> Full Adder1/2(Y)
  AND9/1 -> Full Adder1/1(X)
  Half Adder1/2(Carry) -> Full Adder1/3(Z)
  Full Adder/2(C) -> Full Adder2/3(Z)
  Full Adder1/1(S) -> Full Adder2/2(Y)
  AND10/1 -> Full Adder2/1(X)
  Full Adder2/1(S) -> Bit-3/1
  AND11/1 -> Full Adder3/2(Y)
  AND12/1 -> Full Adder3/1(X)
  Half Adder2/2(Carry) -> Full Adder3/3(Z)
  Full Adder1/2(C) -> Full Adder4/3(Z)
  Full Adder3/1(S) -> Full Adder4/2(Y)
  AND13/1 -> Full Adder4/1(X)
  Full Adder4/1(S) -> Half Adder3/1(A)
  Full Adder2/2(C) -> Half Adder3/2(B)
  A1/1 -> AND11/1, AND8/1, AND5/1, AND2/1
  AND15/1 -> Full Adder5/1(X)
  AND14/1 -> Full Adder5/2(Y)
  Full Adder3/2(C) -> Full Adder5/3(Z)
  Full Adder4/2(C) -> Full Adder6/2(Y)
  Half Adder3/1(Sum) -> Bit-4/1
  Half Adder3/2(Carry) -> Full Adder6/3(Z)
  Full Adder5/1(S) -> Full Adder6/1(X)
  Full Adder6/1(S) -> Bit-5/1
  Full Adder5/2(C) -> Full Adder7/2(Y)
  Full Adder6/2(C) -> Full Adder7/3(Z)
  AND16/1 -> Full Adder7/1(X)
  Full Adder7/1(S) -> Bit-6/1
  Full Adder7/2(C) -> Bit-7/1

== system sequentialProcessorNarenKolli/8-Bit_Processor /8-Bit_Multiplier/First 8-Bit_Adder ==
  A : Inport  OutDataTypeStr=uint8
  B : Inport  Port=2  OutDataTypeStr=uint8
  Bit Concat : hdlsllib/Logic and Bit Operations/Bit Concat  numInputs=8
      settings: SourceProductName=HDL Coder  SourceProductBaseCode=HD
  Constant2 : Constant  Value=0  OutDataTypeStr=boolean
  Full Adder : Subsystem
  Full Adder1 : Subsystem
  Full Adder2 : Subsystem
  Full Adder3 : Subsystem
  Full Adder4 : Subsystem
  Full Adder5 : Subsystem
  Full Adder6 : Subsystem
  Full Adder7 : Subsystem
  Slicer : Subsystem
  Slicer1 : Subsystem
  Sum : Outport  OutDataTypeStr=uint8
  wires:
  Slicer/3(Y5) -> Full Adder5/1(X)
  Slicer1/7(Y1) -> Full Adder1/2(Y)
  Full Adder7/1(S) -> Bit Concat/1
  Slicer/1(Y7) -> Full Adder7/1(X)
  Full Adder6/1(S) -> Bit Concat/2
  Slicer/2(Y6) -> Full Adder6/1(X)
  Slicer/7(Y1) -> Full Adder1/1(X)
  Slicer1/3(Y5) -> Full Adder5/2(Y)
  Full Adder2/1(S) -> Bit Concat/6
  Slicer1/4(Y4) -> Full Adder4/2(Y)
  Full Adder4/2(C) -> Full Adder5/3(Z)
  Full Adder1/2(C) -> Full Adder2/3(Z)
  Slicer/6(Y2) -> Full Adder2/1(X)
  B/1 -> Slicer1/1(X)
  Slicer/8(Y0) -> Full Adder/1(X)
  Full Adder/1(S) -> Bit Concat/8
  Full Adder1/1(S) -> Bit Concat/7
  Slicer1/1(Y7) -> Full Adder7/2(Y)
  Full Adder4/1(S) -> Bit Concat/4
  Full Adder3/1(S) -> Bit Concat/5
  Full Adder5/2(C) -> Full Adder6/3(Z)
  Slicer1/8(Y0) -> Full Adder/2(Y)
  Slicer1/2(Y6) -> Full Adder6/2(Y)
  Full Adder5/1(S) -> Bit Concat/3
  Full Adder/2(C) -> Full Adder1/3(Z)
  Constant2/1 -> Full Adder/3(Z)
  Full Adder6/2(C) -> Full Adder7/3(Z)
  Full Adder3/2(C) -> Full Adder4/3(Z)
  Bit Concat/1 -> Sum/1
  Slicer1/6(Y2) -> Full Adder2/2(Y)
  Slicer1/5(Y3) -> Full Adder3/2(Y)
  A/1 -> Slicer/1(X)
  Full Adder2/2(C) -> Full Adder3/3(Z)
  Slicer/4(Y4) -> Full Adder4/1(X)
  Slicer/5(Y3) -> Full Adder3/1(X)

== system sequentialProcessorNarenKolli/8-Bit_Processor /8-Bit_Multiplier/First Slicer  ==
  X : Inport  OutDataTypeStr=uint8  SampleTime=1
  Bit Slice : hdlsllib/Logic and Bit Operations/Bit Slice  lidx=7  ridx=7
  Bit Slice1 : hdlsllib/Logic and Bit Operations/Bit Slice  lidx=6  ridx=6
  Bit Slice2 : hdlsllib/Logic and Bit Operations/Bit Slice  lidx=5  ridx=5
  Bit Slice3 : hdlsllib/Logic and Bit Operations/Bit Slice  lidx=4  ridx=4
  Bit Slice4 : hdlsllib/Logic and Bit Operations/Bit Slice  lidx=3  ridx=3
  Bit Slice5 : hdlsllib/Logic and Bit Operations/Bit Slice  lidx=2  ridx=2
  Bit Slice6 : hdlsllib/Logic and Bit Operations/Bit Slice  lidx=1  ridx=1
  Bit Slice7 : hdlsllib/Logic and Bit Operations/Bit Slice  lidx=0  ridx=0
  Data Type Conversion{,1..7} (8 alike) : DataTypeConversion  OutDataTypeStr=boolean
  Y7 : Outport  OutDataTypeStr=boolean
  Y6 : Outport  Port=2  OutDataTypeStr=boolean
  Y5 : Outport  Port=3  OutDataTypeStr=boolean
  Y4 : Outport  Port=4  OutDataTypeStr=boolean
  Y3 : Outport  Port=5  OutDataTypeStr=boolean
  Y2 : Outport  Port=6  OutDataTypeStr=boolean
  Y1 : Outport  Port=7  OutDataTypeStr=boolean
  Y0 : Outport  Port=8  OutDataTypeStr=boolean
  wires:
  Data Type Conversion4/1 -> Y4/1
  Bit Slice3/1 -> Data Type Conversion4/1
  X/1 -> Bit Slice3/1, Bit Slice2/1, Bit Slice1/1, Bit Slice/1, Bit Slice4/1, Bit Slice5/1, Bit Slice6/1, Bit Slice7/1
  Bit Slice1/1 -> Data Type Conversion6/1
  Data Type Conversion1/1 -> Y1/1
  Bit Slice6/1 -> Data Type Conversion1/1
  Bit Slice5/1 -> Data Type Conversion2/1
  Bit Slice2/1 -> Data Type Conversion5/1
  Data Type Conversion/1 -> Y0/1
  Bit Slice4/1 -> Data Type Conversion3/1
  Bit Slice/1 -> Data Type Conversion7/1
  Data Type Conversion7/1 -> Y7/1
  Bit Slice7/1 -> Data Type Conversion/1
  Data Type Conversion3/1 -> Y3/1
  Data Type Conversion5/1 -> Y5/1
  Data Type Conversion6/1 -> Y6/1
  Data Type Conversion2/1 -> Y2/1

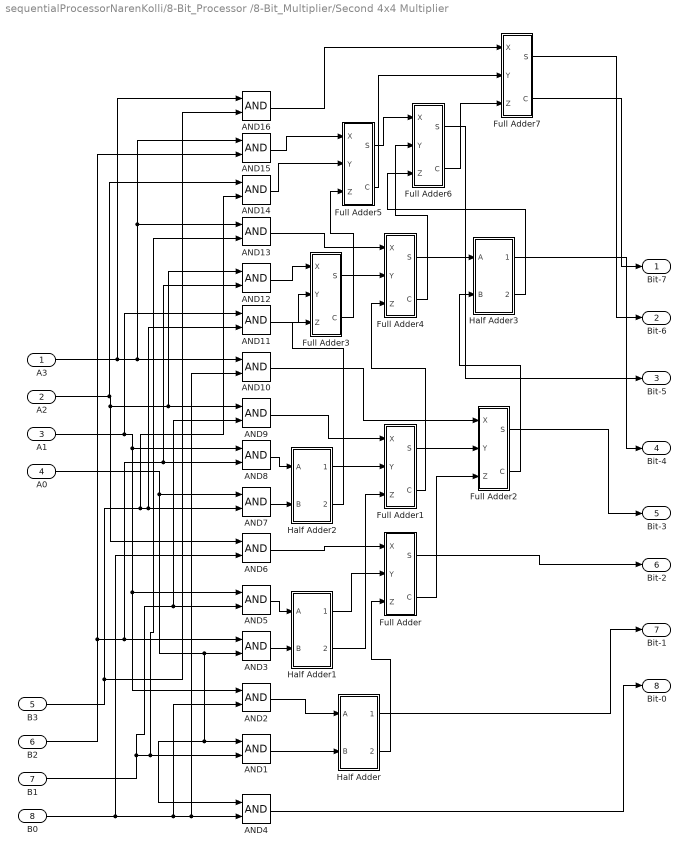
== system sequentialProcessorNarenKolli/8-Bit_Processor /8-Bit_Multiplier/Second 4x4 Multiplier ==
  A3 : Inport  OutDataTypeStr=boolean
  A2 : Inport  Port=2  OutDataTypeStr=boolean
  A1 : Inport  Port=3  OutDataTypeStr=boolean
  A0 : Inport  Port=4  OutDataTypeStr=boolean
  B3 : Inport  Port=5  OutDataTypeStr=boolean
  B2 : Inport  Port=6  OutDataTypeStr=boolean
  B1 : Inport  Port=7  OutDataTypeStr=boolean
  B0 : Inport  Port=8  OutDataTypeStr=boolean
  AND{1..16} (16 alike) : Logic  AllPortsSameDT=off  OutDataTypeStr=boolean
  Full Adder : Subsystem
  Full Adder1 : Subsystem
  Full Adder2 : Subsystem
  Full Adder3 : Subsystem
  Full Adder4 : Subsystem
  Full Adder5 : Subsystem
  Full Adder6 : Subsystem
  Full Adder7 : Subsystem
  Half Adder : Subsystem
  Half Adder1 : Subsystem
  Half Adder2 : Subsystem
  Half Adder3 : Subsystem
  Bit-7 : Outport  OutDataTypeStr=boolean
  Bit-6 : Outport  Port=2  OutDataTypeStr=boolean
  Bit-5 : Outport  Port=3  OutDataTypeStr=boolean
  Bit-4 : Outport  Port=4  OutDataTypeStr=boolean
  Bit-3 : Outport  Port=5  OutDataTypeStr=boolean
  Bit-2 : Outport  Port=6  OutDataTypeStr=boolean
  Bit-1 : Outport  Port=7  OutDataTypeStr=boolean
  Bit-0 : Outport  Port=8  OutDataTypeStr=boolean
  wires:
  AND4/1 -> Bit-0/1
  A0/1 -> AND7/1, AND3/2, AND4/1, AND1/1
  B0/1 -> AND6/2, AND10/2, AND4/2, AND2/2
  AND2/1 -> Half Adder/1(A)
  AND1/1 -> Half Adder/2(B)
  Half Adder/1(Sum) -> Bit-1/1
  B2/1 -> AND15/2, AND12/2, AND8/2, AND3/1
  AND3/1 -> Half Adder1/2(B)
  AND5/1 -> Half Adder1/1(A)
  A2/1 -> AND14/1, AND12/1, AND9/1, AND6/1
  Half Adder/2(Carry) -> Full Adder/3(Z)
  Half Adder1/1(Sum) -> Full Adder/2(Y)
  AND6/1 -> Full Adder/1(X)
  Full Adder/1(S) -> Bit-2/1
  B3/1 -> AND16/2, AND14/2, AND11/2, AND7/2
  B1/1 -> AND9/2, AND5/2, AND13/2, AND1/2
  A3/1 -> AND16/1, AND15/1, AND13/1, AND10/1
  AND7/1 -> Half Adder2/2(B)
  AND8/1 -> Half Adder2/1(A)
  Half Adder2/1(Sum) -> Full Adder1/2(Y)
  AND9/1 -> Full Adder1/1(X)
  Half Adder1/2(Carry) -> Full Adder1/3(Z)
  Full Adder/2(C) -> Full Adder2/3(Z)
  Full Adder1/1(S) -> Full Adder2/2(Y)
  AND10/1 -> Full Adder2/1(X)
  Full Adder2/1(S) -> Bit-3/1
  AND11/1 -> Full Adder3/2(Y)
  AND12/1 -> Full Adder3/1(X)
  Half Adder2/2(Carry) -> Full Adder3/3(Z)
  Full Adder1/2(C) -> Full Adder4/3(Z)
  Full Adder3/1(S) -> Full Adder4/2(Y)
  AND13/1 -> Full Adder4/1(X)
  Full Adder4/1(S) -> Half Adder3/1(A)
  Full Adder2/2(C) -> Half Adder3/2(B)
  A1/1 -> AND11/1, AND8/1, AND5/1, AND2/1
  AND15/1 -> Full Adder5/1(X)
  AND14/1 -> Full Adder5/2(Y)
  Full Adder3/2(C) -> Full Adder5/3(Z)
  Full Adder4/2(C) -> Full Adder6/2(Y)
  Half Adder3/1(Sum) -> Bit-4/1
  Half Adder3/2(Carry) -> Full Adder6/3(Z)
  Full Adder5/1(S) -> Full Adder6/1(X)
  Full Adder6/1(S) -> Bit-5/1
  Full Adder5/2(C) -> Full Adder7/2(Y)
  Full Adder6/2(C) -> Full Adder7/3(Z)
  AND16/1 -> Full Adder7/1(X)
  Full Adder7/1(S) -> Bit-6/1
  Full Adder7/2(C) -> Bit-7/1

== system sequentialProcessorNarenKolli/8-Bit_Processor /8-Bit_Multiplier/Second 8-Bit_Adder1 ==
  A : Inport  OutDataTypeStr=uint8
  B : Inport  Port=2  OutDataTypeStr=uint8
  Bit Concat : hdlsllib/Logic and Bit Operations/Bit Concat  numInputs=8
      settings: SourceProductName=HDL Coder  SourceProductBaseCode=HD
  Constant2 : Constant  Value=0  OutDataTypeStr=boolean
  Full Adder : Subsystem
  Full Adder1 : Subsystem
  Full Adder2 : Subsystem
  Full Adder3 : Subsystem
  Full Adder4 : Subsystem
  Full Adder5 : Subsystem
  Full Adder6 : Subsystem
  Full Adder7 : Subsystem
  Slicer : Subsystem
  Slicer1 : Subsystem
  Sum : Outport  OutDataTypeStr=uint8
  wires:
  Slicer/3(Y5) -> Full Adder5/1(X)
  Slicer1/7(Y1) -> Full Adder1/2(Y)
  Full Adder7/1(S) -> Bit Concat/1
  Slicer/1(Y7) -> Full Adder7/1(X)
  Full Adder6/1(S) -> Bit Concat/2
  Slicer/2(Y6) -> Full Adder6/1(X)
  Slicer/7(Y1) -> Full Adder1/1(X)
  Slicer1/3(Y5) -> Full Adder5/2(Y)
  Full Adder2/1(S) -> Bit Concat/6
  Slicer1/4(Y4) -> Full Adder4/2(Y)
  Full Adder4/2(C) -> Full Adder5/3(Z)
  Full Adder1/2(C) -> Full Adder2/3(Z)
  Slicer/6(Y2) -> Full Adder2/1(X)
  B/1 -> Slicer1/1(X)
  Slicer/8(Y0) -> Full Adder/1(X)
  Full Adder/1(S) -> Bit Concat/8
  Full Adder1/1(S) -> Bit Concat/7
  Slicer1/1(Y7) -> Full Adder7/2(Y)
  Full Adder4/1(S) -> Bit Concat/4
  Full Adder3/1(S) -> Bit Concat/5
  Full Adder5/2(C) -> Full Adder6/3(Z)
  Slicer1/8(Y0) -> Full Adder/2(Y)
  Slicer1/2(Y6) -> Full Adder6/2(Y)
  Full Adder5/1(S) -> Bit Concat/3
  Full Adder/2(C) -> Full Adder1/3(Z)
  Constant2/1 -> Full Adder/3(Z)
  Full Adder6/2(C) -> Full Adder7/3(Z)
  Full Adder3/2(C) -> Full Adder4/3(Z)
  Bit Concat/1 -> Sum/1
  Slicer1/6(Y2) -> Full Adder2/2(Y)
  Slicer1/5(Y3) -> Full Adder3/2(Y)
  A/1 -> Slicer/1(X)
  Full Adder2/2(C) -> Full Adder3/3(Z)
  Slicer/4(Y4) -> Full Adder4/1(X)
  Slicer/5(Y3) -> Full Adder3/1(X)

== system sequentialProcessorNarenKolli/8-Bit_Processor /8-Bit_Multiplier/Second Slicer ==
  X : Inport  OutDataTypeStr=uint8  SampleTime=1
  Bit Slice : hdlsllib/Logic and Bit Operations/Bit Slice  lidx=7  ridx=7
  Bit Slice1 : hdlsllib/Logic and Bit Operations/Bit Slice  lidx=6  ridx=6
  Bit Slice2 : hdlsllib/Logic and Bit Operations/Bit Slice  lidx=5  ridx=5
  Bit Slice3 : hdlsllib/Logic and Bit Operations/Bit Slice  lidx=4  ridx=4
  Bit Slice4 : hdlsllib/Logic and Bit Operations/Bit Slice  lidx=3  ridx=3
  Bit Slice5 : hdlsllib/Logic and Bit Operations/Bit Slice  lidx=2  ridx=2
  Bit Slice6 : hdlsllib/Logic and Bit Operations/Bit Slice  lidx=1  ridx=1
  Bit Slice7 : hdlsllib/Logic and Bit Operations/Bit Slice  lidx=0  ridx=0
  Data Type Conversion{,1..7} (8 alike) : DataTypeConversion  OutDataTypeStr=boolean
  Y7 : Outport  OutDataTypeStr=boolean
  Y6 : Outport  Port=2  OutDataTypeStr=boolean
  Y5 : Outport  Port=3  OutDataTypeStr=boolean
  Y4 : Outport  Port=4  OutDataTypeStr=boolean
  Y3 : Outport  Port=5  OutDataTypeStr=boolean
  Y2 : Outport  Port=6  OutDataTypeStr=boolean
  Y1 : Outport  Port=7  OutDataTypeStr=boolean
  Y0 : Outport  Port=8  OutDataTypeStr=boolean
  wires:
  Data Type Conversion4/1 -> Y4/1
  Bit Slice3/1 -> Data Type Conversion4/1
  X/1 -> Bit Slice3/1, Bit Slice2/1, Bit Slice1/1, Bit Slice/1, Bit Slice4/1, Bit Slice5/1, Bit Slice6/1, Bit Slice7/1
  Bit Slice1/1 -> Data Type Conversion6/1
  Data Type Conversion1/1 -> Y1/1
  Bit Slice6/1 -> Data Type Conversion1/1
  Bit Slice5/1 -> Data Type Conversion2/1
  Bit Slice2/1 -> Data Type Conversion5/1
  Data Type Conversion/1 -> Y0/1
  Bit Slice4/1 -> Data Type Conversion3/1
  Bit Slice/1 -> Data Type Conversion7/1
  Data Type Conversion7/1 -> Y7/1
  Bit Slice7/1 -> Data Type Conversion/1
  Data Type Conversion3/1 -> Y3/1
  Data Type Conversion5/1 -> Y5/1
  Data Type Conversion6/1 -> Y6/1
  Data Type Conversion2/1 -> Y2/1

== system sequentialProcessorNarenKolli/8-Bit_Processor /8-Bit_Multiplier/Third Slicer ==
  X : Inport  OutDataTypeStr=uint8  SampleTime=1
  Bit Slice : hdlsllib/Logic and Bit Operations/Bit Slice  lidx=7  ridx=7
  Bit Slice1 : hdlsllib/Logic and Bit Operations/Bit Slice  lidx=6  ridx=6
  Bit Slice2 : hdlsllib/Logic and Bit Operations/Bit Slice  lidx=5  ridx=5
  Bit Slice3 : hdlsllib/Logic and Bit Operations/Bit Slice  lidx=4  ridx=4
  Bit Slice4 : hdlsllib/Logic and Bit Operations/Bit Slice  lidx=3  ridx=3
  Bit Slice5 : hdlsllib/Logic and Bit Operations/Bit Slice  lidx=2  ridx=2
  Bit Slice6 : hdlsllib/Logic and Bit Operations/Bit Slice  lidx=1  ridx=1
  Bit Slice7 : hdlsllib/Logic and Bit Operations/Bit Slice  lidx=0  ridx=0
  Data Type Conversion{,1..7} (8 alike) : DataTypeConversion  OutDataTypeStr=boolean
  Y7 : Outport  OutDataTypeStr=boolean
  Y6 : Outport  Port=2  OutDataTypeStr=boolean
  Y5 : Outport  Port=3  OutDataTypeStr=boolean
  Y4 : Outport  Port=4  OutDataTypeStr=boolean
  Y3 : Outport  Port=5  OutDataTypeStr=boolean
  Y2 : Outport  Port=6  OutDataTypeStr=boolean
  Y1 : Outport  Port=7  OutDataTypeStr=boolean
  Y0 : Outport  Port=8  OutDataTypeStr=boolean
  wires:
  Data Type Conversion4/1 -> Y4/1
  Bit Slice3/1 -> Data Type Conversion4/1
  X/1 -> Bit Slice3/1, Bit Slice2/1, Bit Slice1/1, Bit Slice/1, Bit Slice4/1, Bit Slice5/1, Bit Slice6/1, Bit Slice7/1
  Bit Slice1/1 -> Data Type Conversion6/1
  Data Type Conversion1/1 -> Y1/1
  Bit Slice6/1 -> Data Type Conversion1/1
  Bit Slice5/1 -> Data Type Conversion2/1
  Bit Slice2/1 -> Data Type Conversion5/1
  Data Type Conversion/1 -> Y0/1
  Bit Slice4/1 -> Data Type Conversion3/1
  Bit Slice/1 -> Data Type Conversion7/1
  Data Type Conversion7/1 -> Y7/1
  Bit Slice7/1 -> Data Type Conversion/1
  Data Type Conversion3/1 -> Y3/1
  Data Type Conversion5/1 -> Y5/1
  Data Type Conversion6/1 -> Y6/1
  Data Type Conversion2/1 -> Y2/1

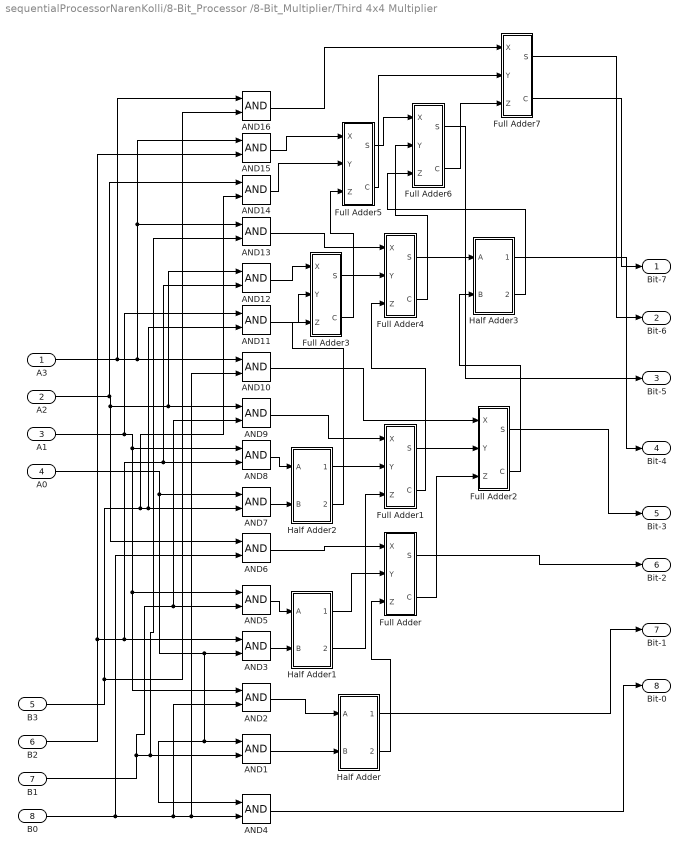
== system sequentialProcessorNarenKolli/8-Bit_Processor /8-Bit_Multiplier/Third 4x4 Multiplier ==
  A3 : Inport  OutDataTypeStr=boolean
  A2 : Inport  Port=2  OutDataTypeStr=boolean
  A1 : Inport  Port=3  OutDataTypeStr=boolean
  A0 : Inport  Port=4  OutDataTypeStr=boolean
  B3 : Inport  Port=5  OutDataTypeStr=boolean
  B2 : Inport  Port=6  OutDataTypeStr=boolean
  B1 : Inport  Port=7  OutDataTypeStr=boolean
  B0 : Inport  Port=8  OutDataTypeStr=boolean
  AND{1..16} (16 alike) : Logic  AllPortsSameDT=off  OutDataTypeStr=boolean
  Full Adder : Subsystem
  Full Adder1 : Subsystem
  Full Adder2 : Subsystem
  Full Adder3 : Subsystem
  Full Adder4 : Subsystem
  Full Adder5 : Subsystem
  Full Adder6 : Subsystem
  Full Adder7 : Subsystem
  Half Adder : Subsystem
  Half Adder1 : Subsystem
  Half Adder2 : Subsystem
  Half Adder3 : Subsystem
  Bit-7 : Outport  OutDataTypeStr=boolean
  Bit-6 : Outport  Port=2  OutDataTypeStr=boolean
  Bit-5 : Outport  Port=3  OutDataTypeStr=boolean
  Bit-4 : Outport  Port=4  OutDataTypeStr=boolean
  Bit-3 : Outport  Port=5  OutDataTypeStr=boolean
  Bit-2 : Outport  Port=6  OutDataTypeStr=boolean
  Bit-1 : Outport  Port=7  OutDataTypeStr=boolean
  Bit-0 : Outport  Port=8  OutDataTypeStr=boolean
  wires:
  AND4/1 -> Bit-0/1
  A0/1 -> AND7/1, AND3/2, AND4/1, AND1/1
  B0/1 -> AND6/2, AND10/2, AND4/2, AND2/2
  AND2/1 -> Half Adder/1(A)
  AND1/1 -> Half Adder/2(B)
  Half Adder/1(Sum) -> Bit-1/1
  B2/1 -> AND15/2, AND12/2, AND8/2, AND3/1
  AND3/1 -> Half Adder1/2(B)
  AND5/1 -> Half Adder1/1(A)
  A2/1 -> AND14/1, AND12/1, AND9/1, AND6/1
  Half Adder/2(Carry) -> Full Adder/3(Z)
  Half Adder1/1(Sum) -> Full Adder/2(Y)
  AND6/1 -> Full Adder/1(X)
  Full Adder/1(S) -> Bit-2/1
  B3/1 -> AND16/2, AND14/2, AND11/2, AND7/2
  B1/1 -> AND9/2, AND5/2, AND13/2, AND1/2
  A3/1 -> AND16/1, AND15/1, AND13/1, AND10/1
  AND7/1 -> Half Adder2/2(B)
  AND8/1 -> Half Adder2/1(A)
  Half Adder2/1(Sum) -> Full Adder1/2(Y)
  AND9/1 -> Full Adder1/1(X)
  Half Adder1/2(Carry) -> Full Adder1/3(Z)
  Full Adder/2(C) -> Full Adder2/3(Z)
  Full Adder1/1(S) -> Full Adder2/2(Y)
  AND10/1 -> Full Adder2/1(X)
  Full Adder2/1(S) -> Bit-3/1
  AND11/1 -> Full Adder3/2(Y)
  AND12/1 -> Full Adder3/1(X)
  Half Adder2/2(Carry) -> Full Adder3/3(Z)
  Full Adder1/2(C) -> Full Adder4/3(Z)
  Full Adder3/1(S) -> Full Adder4/2(Y)
  AND13/1 -> Full Adder4/1(X)
  Full Adder4/1(S) -> Half Adder3/1(A)
  Full Adder2/2(C) -> Half Adder3/2(B)
  A1/1 -> AND11/1, AND8/1, AND5/1, AND2/1
  AND15/1 -> Full Adder5/1(X)
  AND14/1 -> Full Adder5/2(Y)
  Full Adder3/2(C) -> Full Adder5/3(Z)
  Full Adder4/2(C) -> Full Adder6/2(Y)
  Half Adder3/1(Sum) -> Bit-4/1
  Half Adder3/2(Carry) -> Full Adder6/3(Z)
  Full Adder5/1(S) -> Full Adder6/1(X)
  Full Adder6/1(S) -> Bit-5/1
  Full Adder5/2(C) -> Full Adder7/2(Y)
  Full Adder6/2(C) -> Full Adder7/3(Z)
  AND16/1 -> Full Adder7/1(X)
  Full Adder7/1(S) -> Bit-6/1
  Full Adder7/2(C) -> Bit-7/1

== system sequentialProcessorNarenKolli/8-Bit_Processor /8-Bit_Subtractor/Full Adder 0 ==
  X : Inport
  Y : Inport  Port=2
  Z : Inport  Port=3
  Half Adder : Subsystem
  Half Adder1 : Subsystem
  OR : Logic  Operator=OR  AllPortsSameDT=off  OutDataTypeStr=boolean
  S : Outport
  C : Outport  Port=2
  wires:
  Half Adder/2(Carry) -> OR/2
  OR/1 -> C/1
  Z/1 -> Half Adder1/2(B)
  X/1 -> Half Adder/1(A)
  Half Adder1/1(Sum) -> S/1
  Half Adder/1(Sum) -> Half Adder1/1(A)
  Y/1 -> Half Adder/2(B)
  Half Adder1/2(Carry) -> OR/1

== system sequentialProcessorNarenKolli/8-Bit_Processor /8-Bit_Subtractor/Full Adder 1 ==
  X : Inport
  Y : Inport  Port=2
  Z : Inport  Port=3
  Half Adder : Subsystem
  Half Adder1 : Subsystem
  OR : Logic  Operator=OR  AllPortsSameDT=off  OutDataTypeStr=boolean
  S : Outport
  C : Outport  Port=2
  wires:
  Half Adder/2(Carry) -> OR/2
  OR/1 -> C/1
  Z/1 -> Half Adder1/2(B)
  X/1 -> Half Adder/1(A)
  Half Adder1/1(Sum) -> S/1
  Half Adder/1(Sum) -> Half Adder1/1(A)
  Y/1 -> Half Adder/2(B)
  Half Adder1/2(Carry) -> OR/1

== system sequentialProcessorNarenKolli/8-Bit_Processor /8-Bit_Subtractor/Full Adder 2  ==
  X : Inport
  Y : Inport  Port=2
  Z : Inport  Port=3
  Half Adder : Subsystem
  Half Adder1 : Subsystem
  OR : Logic  Operator=OR  AllPortsSameDT=off  OutDataTypeStr=boolean
  S : Outport
  C : Outport  Port=2
  wires:
  Half Adder/2(Carry) -> OR/2
  OR/1 -> C/1
  Z/1 -> Half Adder1/2(B)
  X/1 -> Half Adder/1(A)
  Half Adder1/1(Sum) -> S/1
  Half Adder/1(Sum) -> Half Adder1/1(A)
  Y/1 -> Half Adder/2(B)
  Half Adder1/2(Carry) -> OR/1

== system sequentialProcessorNarenKolli/8-Bit_Processor /8-Bit_Subtractor/Full Adder 3  ==
  X : Inport
  Y : Inport  Port=2
  Z : Inport  Port=3
  Half Adder : Subsystem
  Half Adder1 : Subsystem
  OR : Logic  Operator=OR  AllPortsSameDT=off  OutDataTypeStr=boolean
  S : Outport
  C : Outport  Port=2
  wires:
  Half Adder/2(Carry) -> OR/2
  OR/1 -> C/1
  Z/1 -> Half Adder1/2(B)
  X/1 -> Half Adder/1(A)
  Half Adder1/1(Sum) -> S/1
  Half Adder/1(Sum) -> Half Adder1/1(A)
  Y/1 -> Half Adder/2(B)
  Half Adder1/2(Carry) -> OR/1

== system sequentialProcessorNarenKolli/8-Bit_Processor /8-Bit_Subtractor/Full Adder 4 ==
  X : Inport
  Y : Inport  Port=2
  Z : Inport  Port=3
  Half Adder : Subsystem
  Half Adder1 : Subsystem
  OR : Logic  Operator=OR  AllPortsSameDT=off  OutDataTypeStr=boolean
  S : Outport
  C : Outport  Port=2
  wires:
  Half Adder/2(Carry) -> OR/2
  OR/1 -> C/1
  Z/1 -> Half Adder1/2(B)
  X/1 -> Half Adder/1(A)
  Half Adder1/1(Sum) -> S/1
  Half Adder/1(Sum) -> Half Adder1/1(A)
  Y/1 -> Half Adder/2(B)
  Half Adder1/2(Carry) -> OR/1

== system sequentialProcessorNarenKolli/8-Bit_Processor /8-Bit_Subtractor/Full Adder 5  ==
  X : Inport
  Y : Inport  Port=2
  Z : Inport  Port=3
  Half Adder : Subsystem
  Half Adder1 : Subsystem
  OR : Logic  Operator=OR  AllPortsSameDT=off  OutDataTypeStr=boolean
  S : Outport
  C : Outport  Port=2
  wires:
  Half Adder/2(Carry) -> OR/2
  OR/1 -> C/1
  Z/1 -> Half Adder1/2(B)
  X/1 -> Half Adder/1(A)
  Half Adder1/1(Sum) -> S/1
  Half Adder/1(Sum) -> Half Adder1/1(A)
  Y/1 -> Half Adder/2(B)
  Half Adder1/2(Carry) -> OR/1
